simulink library "SimFly_System"  (R2015b)
settings: Solver=VariableStepAuto  StartTime=0.0  StopTime=10.0  RelTol=1e-3
settings Model: Creator=mocherma  LastModifiedBy=mocherma

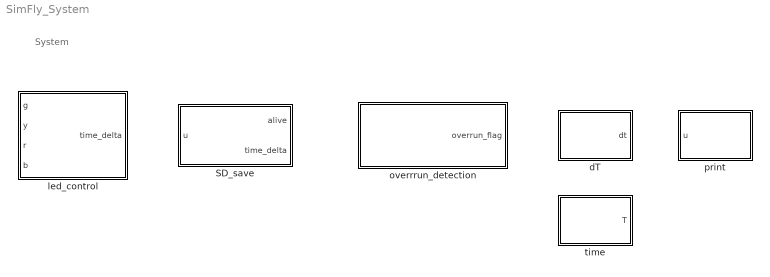
== system SimFly_System ==
  note: System
  SD_save : MATLAB Function  TreatAsAtomicUnit=on  mask(SimFly SD LOG){save_rate=60, sd_sample_time=-1}
      mask prompts: save_rate "Save Rate"; sd_sample_time "Sample Time"
      mask help:
      | Saves data to SD-Card
      | Card must be FAT16/32
      | Sample Time should not be -1 in this case
      | Save Rate =  Cycle in seconds in which the data should be saved (reduces execution time)
  dT : MATLAB Function  TreatAsAtomicUnit=on  mask(SimFly Delta Time){}
      mask help: Returns delta time
  led_control : MATLAB Function  TreatAsAtomicUnit=on  mask(SimFly LED){}
      mask help:
      | Input 1 for LED flashing
      |
      | Green   (Pin47)
      |
      | Yellow  (Pin48)
      |
      | Red     (Pin49)
      |
      | Blue    (Pin50)
  overrrun_detection : MATLAB Function  TreatAsAtomicUnit=on  mask(SimFly Overrun Detection){sample_time=0}
      mask prompts: sample_time "Sample Time"
      mask help:
      | Manual overrun detection.
      | Enter sampe time at which model is running.
      | Output: true if actual sample time is larger than specified sample time.
      | Do not enter -1 in sample time!
  print : MATLAB Function  TreatAsAtomicUnit=on
  time : MATLAB Function  TreatAsAtomicUnit=on

== matlab function SimFly_System/time ==
  data: T output
function T = time_s()
%PURPOSE: Function to get the time since startup
%AUTHOR: Marcell Mocher
%DATE: 10.6.2016
%VERSION: 0.1 V Fist build
%Input:
%Outpu: time in s
%Info: This drive requires function call triggered simuluink functions in
% order to work
%Requires:  _get_time

if strcmp(coder.target, 'rtw'),
    time = uint32(0);
    time = coder.ceval('_get_time');
    T = single(time) * 1e-6;
else
    T = single(1);
end

== matlab function SimFly_System/SD_save ==
  settings: updateMethod=DISCRETE  sampleTime=sd_sample_time
  data: alive output; u input; time_delta output; save_rate parameter; sd_sample_time parameter
function [alive,time_delta]  =  sd(u, save_rate, sd_sample_time)
%PURPOSE: Driver for Micro SD with hardware abstraction layer
%AUTHOR: Marcell Mocher
%DATE: 23.6.2016
%VERSION: 0.1 V Fist build
%Input: -
%Output:
%           alive(boolean) = boolean if sd_card is alive
%           time_delta(single) = time needed to execute funtion [us]
%Info: This drive requires function call triggered simuluink functions in
% order to work
%Requires:  _get_time
%           _sd_init
%           _sd_open
%           _sd_close
%           _sd_nl
%           _sd_print_tab

persistent init alive_flag count closed timeout_count

% mask parameters


% set maximum allowed execution time
overflow_time = uint32(5000);  

if sd_sample_time < 1
save_cycles = uint32(10000);
else
save_cycles = uint32(save_rate / sd_sample_time);
end

%save_cycles = uint32(10000); % save_cycles * sample time is the time in which the file is saved 10000





if strcmp(coder.target, 'rtw'),
    
    %Save time for measurement
    time_start = uint32(0);
    time_start = coder.ceval('_get_time');
    
    % initialization function
    if isempty(init)
        init = 1;
        count = uint32(0);
        closed = false;
        alive_flag = false;
        timeout_count = uint8(0);
        alive_flag = coder.ceval('_sd_init');
    end
    
    % Only save params when sd card is healthy
    if alive_flag == true
        
        % See if file was closed in the last step
        if closed == true
            alive_flag = coder.ceval('_sd_open');
            closed = false;
            count = uint32(0);
        end
        
        % This is the actual printing part
        
        time_now = uint32(0);
        time_now = coder.ceval('_get_time');
        coder.ceval('_sd_print_tab',double(time_now),uint8(0));
        
        for i = 1:numel(u)
            coder.ceval('_sd_print_tab',u(i),uint8(4));
        end
        coder.ceval('_sd_nl');
        
        % Routin to save data to file
        if count > save_cycles
            coder.ceval('_sd_close');
            closed = true;
        end
        
        count = count + 1;
        
    end
    
    % Calculate execution time
    time_end = uint32(0);
    time_end = coder.ceval('_get_time');
    time_delta = time_end - time_start;
    % See if there was an overflow after 5 overflows set alive flag false
    if time_delta > overflow_time
        timeout_count = timeout_count + 1;
        if(timeout_count > 5)
            alive_flag = false;
        end
    else
        timeout_count = uint8(0);
    end
    
    alive = alive_flag;
    %Sim mode only
else
    alive = true;
    time_delta = uint32(1);
end

end

== matlab function SimFly_System/led_control ==
  data: g input; y input; r input; b input; time_delta output
function time_delta = led(g,y,r,b)
%PURPOSE: Driver for LEDs with hardware abstraction layer
%AUTHOR: Marcell Mocher
%DATE: 10.6.2016
%VERSION: 0.1 V Fist build
%Input:    g,y,r,b booleans for LEDs
%Output:   time_delta(single) = time needed to execute funtion [us]
%Info: This drive requires function call triggered simuluink functions in
% order to work
%Requires:  _get_time
%           _led_init
%           _led_on_off

persistent init_flag

if strcmp(coder.target, 'rtw'),
    
    time_start = uint32(0);
    time_start = coder.ceval('_get_time');
    
    if isempty(init_flag)
        init_flag = true;
        coder.ceval('_led_init');
    end
    
    coder.ceval('_led_on_off',uint8(0),g);
    coder.ceval('_led_on_off',uint8(1),y);
    coder.ceval('_led_on_off',uint8(2),r);
    coder.ceval('_led_on_off',uint8(3),b);
    
    time_end = uint32(0);
    time_end = coder.ceval('_get_time');
    time_delta = time_end - time_start;
else
    time_delta = uint32(0);
end
end

== matlab function SimFly_System/print ==
  data: u input
function print(u)
%PURPOSE: Example Driver for Serial printing with hardware abstraction layer
%AUTHOR: Marcell Mocher
%DATE: 10.6.2016
%VERSION: 0.1 V Fist build
%Input: Array to print on the serial port
%Info: This drive requires function call triggered simuluink functions in
% order to work
%Requires:  _get_time
%           _serial_init
%           _serial_print
%           _serial_write

persistent init_flag
 
if strcmp(coder.target, 'rtw'),
    
    time_start = uint32(0);
    time_start = coder.ceval('_get_time');
    
    
   if isempty(init_flag)
      init_flag = true;      
      coder.ceval('_serial_init',uint8(0),uint32(250000));
   end
    
   coder.ceval('_serial_print',uint8(0),double(time_start));
   coder.ceval('_serial_write',uint8(0),uint8(32));
   
   for i = 1:numel(u)
        coder.ceval('_serial_print',uint8(0),double(u(i)));
        coder.ceval('_serial_write',uint8(0),uint8(32));
   end
   
    time_end = uint32(0);
    time_end = coder.ceval('_get_time');
    time_delta = time_end - time_start;
    %coder.ceval('_serial_print',uint8(0),double(time_delta));

    coder.ceval('_serial_write',uint8(0),uint8(10));
end

== matlab function SimFly_System/overrrun_detection ==
  data: overrun_flag output; sample_time parameter single
function overrun_flag = overrun(sample_time)
%#codegen
persistent old_time init_flag

if isempty(init_flag)
    init_flag = true;
    old_time = uint32(0);
end

sample_time = sample_time * 1e6;

if strcmp(coder.target, 'rtw'),
    time = uint32(0);
    time = coder.ceval('_get_time');
    dt = time - old_time;
    old_time = time;
    if dt > sample_time
        overrun_flag = true;
    else
        overrun_flag = false;
    end
else
    overrun_flag = false;
end

== matlab function SimFly_System/dT ==
  data: dt output
function dt = dt()
%#codegen
persistent old_time init_flag

if isempty(init_flag)
    init_flag = true;
    old_time = uint32(0);
end

if strcmp(coder.target, 'rtw'),
    T = uint32(0);
    T = coder.ceval('_get_time');
    delta = T - old_time;
    old_time = T;
    dt = single(delta) * 1e-6;
else
    dt = single(1);
end
